simulink model "LegWithSensors"  (R2017a)
settings: Solver=ode3  StartTime=0.0  StopTime=20  FixedStep=0.01  MaxStep=0.01  RelTol=1e-3  EnableMultiTasking=on
model workspace (MAT data in the model file):
  MCOS : class17 (value not decoded)
values from neighbouring files (symbols this model uses):
  FootLength_cm = 20.0    [Data.sldd]
  FootThickness_cm = 1.0    [Data.sldd]
  GravityVector_ms2 = 0.0 -9.81 0.0    [Data.sldd]
  HipAngleStart_rad = -1.5707963267948966    [Data.sldd]
  KneeActuatorSineAmplitude = 0.78539816339744828    [Data.sldd]
  KneeActuatorSineBias = -1.5707963267948966    [Data.sldd]
  KneeActuatorSineFreq = 2.0    [Data.sldd]
undefined symbols (not defined in the file or in its folder): X, Y, Z
undefined symbols (not defined in the file): BoneDensity_kgm3, FootWidth_cm, LegLength_cm, LegThickness_cm, LegWidth_cm
libraries: sm_lib x34, nesl_utility x22, sharedtransform x4, simulink_extras x1
(part 2 of 2)

== matlab function LegWithSensors/Leg with IMUs/Perfect IMU Upper/Magnetometer Signal Calculation/Rotation Matrix ==
  data: u input; y output
function y = fcn(u)

ax = u(1);
ay = u(2);
az = u(3);

mx = [1  0         0;
      0  cos(ax)   -sin(ax);
      0  sin(ax)  cos(ax)];

my = [cos(ay)   0  sin(ay);
      0         1  0;
      -sin(ay)  0  cos(ay)];

mz = [cos(az)  -sin(az)  0;
      sin(az)  cos(az)   0;
      0        0         1];
  
y = (mz'*my'*mx')';

== matlab function LegWithSensors/Leg with IMUs/Perfect IMU Lower/Magnetometer Signal Calculation/Rotation Matrix ==
  data: u input; y output
function y = fcn(u)

ax = u(1);
ay = u(2);
az = u(3);

mx = [1  0         0;
      0  cos(ax)   -sin(ax);
      0  sin(ax)  cos(ax)];

my = [cos(ay)   0  sin(ay);
      0         1  0;
      -sin(ay)  0  cos(ay)];

mz = [cos(az)  -sin(az)  0;
      sin(az)  cos(az)   0;
      0        0         1];
  
y = (mz'*my'*mx')';
